simulink model "QBot2_SINGLE_ROBOT_FINDFOLLOW_5_clock_working"  (R2014a)
settings: Solver=ode1  StartTime=0.0  StopTime=inf  FixedStep=0.01  RelTol=1e-3
values from neighbouring files (symbols this model uses):
  x = [0 0 0 0 0 0 0 0 0 0 0 0 ... (23417 elements, 23417x1)]    [plot_data.mat]
undefined symbols (not defined in the file or in its folder): HIL, Kinect, qc_get_step_size
libraries: quarc_library x8
settings Model: SimulationMode=external  CovSFcnEnable=on  ExtModeTrigDuration=10000  Creator=drmadill  LastModifiedBy=student
settings SolverCC: PositivePriorityOrder=on
settings DataIOCC: SignalLoggingSaveFormat=ModelDataLogs
settings OptimizationCC: ExpressionDepthLimit=2147483647
settings DebuggingCC: UnderspecifiedInitializationDetection=Classic  FcnCallInpInsideContextMsg=UseLocalSettings  FrameProcessingCompatibilityMsg=error  StateNameClashWarn=warning
settings RTWCC: SystemTargetFile=quarc_linux_duovero.tlc  TemplateMakefile=quarc_linux_duovero_tmf  Description=QUARC Linux DuoVero Target  ProcessScript=quarc_linux_duovero_make_rtw_hook
settings STFCustomTargetCC: TargetLibSuffix=.a  TargetPreCompLibLocation=C:\PROGRA~3\QUARC\lib\2014a\LINUX_~3\release  CPPClassGenCompliant=on  SystemTargetFile=quarc_linux_duovero.tlc
settings GRTTargetCC: TargetLibSuffix=.a  TargetPreCompLibLocation=C:\PROGRA~3\QUARC\lib\2014a\LINUX_~3\release  ParMdlRefBuildCompliant=off  CompOptLevelCompliant=off  CombineOutputUpdateFcns=off  MatFileLogging=off  GRTInterface=on  ExtMode=on  ExtModeMexFile=quarc_comm  ExtModeMexArgs='-w -d /tmp -uri %u', 'tcpip://192.168.2.49:17001'

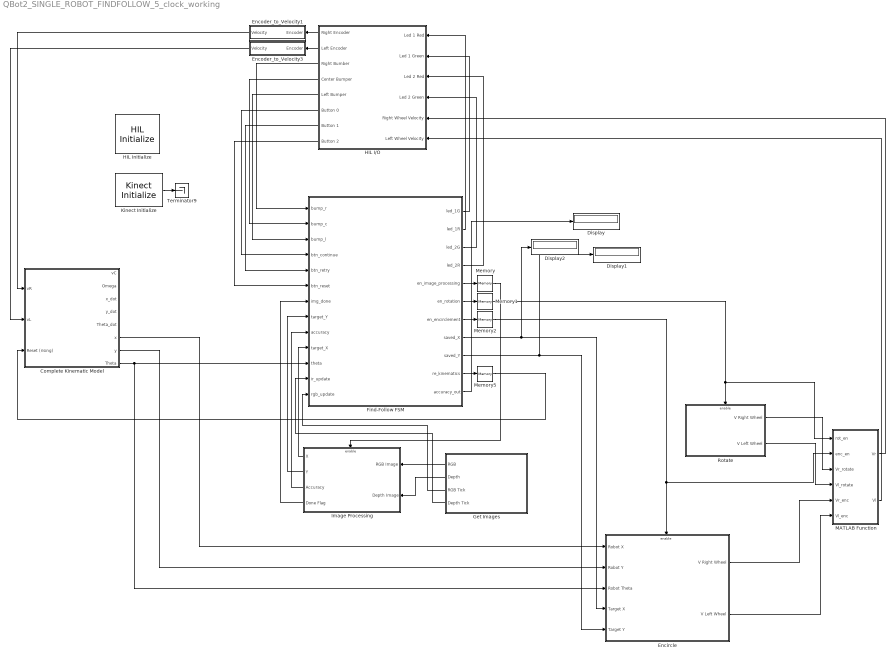
== system QBot2_SINGLE_ROBOT_FINDFOLLOW_5_clock_working ==
  Complete Kinematic Model : Subsystem
  Display : Display
  Display1 : Display
  Display2 : Display
  Encircle : Subsystem  TreatAsAtomicUnit=on
  Encoder_to_Velocity1 : Subsystem
  Encoder_to_Velocity3 : Subsystem
  Find-Follow FSM : Stateflow chart  TreatAsAtomicUnit=on
  Get Images : Subsystem
  HIL I/O : Subsystem
  HIL Initialize : quarc_library/Data Acquisition/Generic/Configuration/HIL Initialize  Priority=-99  object_name=HIL-1  board_type=qbot2  board_number=0  board_options=enc0_dir=0;enc0_filter=1;enc0_a=0;enc0_b=0;enc0_z=1;enc0_reload=0;enc1_dir=0;enc1_filter=1;enc1_a=0;enc1_b=0;enc1_z=1;enc1_reload=0;pwm0_immediate=0;pwm1_immediate=0;pwm2_immediate=0;pwm3_immediate=0;  exclusive=off  active=off  hardware_clocks=[]  clock_modes=[]  initial_clock_frequencies=[]  set_clock_params_at_start=off  set_clock_params_at_switch_in=off  set_clock_frequencies_at_start=off  set_clock_frequencies_at_switch_in=off  analog_input_channels=[0:9]  analog_input_maximums=[5 5 5 5 16.5 3.3 3.3 3.3 3.3]  analog_input_minimums=[0 0 0 0 0 0 0 0 0]  set_analog_input_params_at_start=off  set_analog_input_params_at_switch_in=off  analog_output_channels=[]  analog_output_maximums=[]  analog_output_minimums=[]  initial_analog_outputs=[]  final_analog_outputs=[]  watchdog_analog_outputs=[]  set_analog_output_params_at_start=off  set_analog_output_params_at_switch_in=off  set_analog_outputs_at_start=off  set_analog_outputs_at_switch_in=off  set_analog_outputs_at_terminate=off  set_analog_outputs_at_switch_out=off  set_analog_outputs_on_watchdog=off  digital_input_channels=[8:10 16:18]  digital_output_channels=[11:12 9:10]  digital_output_configuration=[]  initial_digital_outputs=[0]  final_digital_outputs=[0]  watchdog_digital_outputs=[0]  set_digital_output_params_at_start=off  set_digital_output_params_at_switch_in=off  set_digital_outputs_at_start=on  set_digital_outputs_at_switch_in=off  set_digital_outputs_at_terminate=on  set_digital_outputs_at_switch_out=off  set_digital_outputs_on_watchdog=on  encoder_channels=[0:3]  quadrature=[4]  encoder_filter_frequency=[]  initial_encoder_counts=[0]  set_encoder_params_at_start=on  set_encoder_params_at_switch_in=off  set_encoder_counts_at_start=on  set_encoder_counts_at_switch_in=off  pwm_channels=[0:3]  pwm_modes=[0]  pwm_frequency=[20e6/1024]  pwm_configuration=[0]  pwm_alignment=[0]  pwm_polarity=[1]  pwm_leading_deadband=[0]  pwm_trailing_deadband=[0]  initial_pwm_outputs=[0]  final_pwm_outputs=[0]  watchdog_pwm_outputs=[0]  set_pwm_params_at_start=on  set_pwm_params_at_switch_in=off  set_pwm_outputs_at_start=on  set_pwm_outputs_at_switch_in=off  set_pwm_outputs_at_terminate=on  set_pwm_outputs_at_switch_out=off  set_pwm_outputs_on_watchdog=on  other_output_channels=[2000:2001 14000 16000]  initial_other_outputs=[0 0 0 7]  final_other_outputs=[0 0 0 7]  watchdog_other_outputs=[]  set_other_outputs_at_start=on  set_other_outputs_at_switch_in=off  set_other_outputs_at_terminate=on  set_other_outputs_at_switch_out=off  set_other_outputs_on_watchdog=off
  Image Processing : Subsystem
  Kinect Initialize : quarc_library/Multimedia/Kinect Initialize  object_name=Kinect-1  kinect_type=Kinect for XBox 360  identifier=0  sample_time=qc_get_step_size * ceil(0.033 / qc_get_step_size)  active=on
  MATLAB Function : MATLAB Function  TreatAsAtomicUnit=on
  Memory{,1..2,5} (4 alike) : Memory
  Rotate : Subsystem  TreatAsAtomicUnit=on
  Terminator9 : Terminator
  wires:
  Find-Follow FSM/5(en_image_processing) -> Memory/1
  Find-Follow FSM/6(en_rotation) -> Memory1/1
  Find-Follow FSM/7(en_encirclement) -> Memory2/1
  Encoder_to_Velocity3/1(Velocity) -> Complete Kinematic Model/2(vL)
  Encoder_to_Velocity1/1(Velocity) -> Complete Kinematic Model/1(vR)
  Complete Kinematic Model/8(Theta) -> Encircle/3(Robot Theta), Find-Follow FSM/11(theta)
  HIL I/O/1(Right Encoder) -> Encoder_to_Velocity1/1(Encoder)
  HIL I/O/2(Left Encoder) -> Encoder_to_Velocity3/1(Encoder)
  HIL I/O/3(Right Bumber) -> Find-Follow FSM/1(bump_r)
  HIL I/O/4(Center Bumper) -> Find-Follow FSM/2(bump_c)
  HIL I/O/5(Left Bumper) -> Find-Follow FSM/3(bump_l)
  HIL I/O/6(Button 0) -> Find-Follow FSM/4(btn_continue)
  HIL I/O/7(Button 1) -> Find-Follow FSM/5(btn_retry)
  HIL I/O/8(Button 2) -> Find-Follow FSM/6(btn_reset)
  Find-Follow FSM/1(led_1G) -> HIL I/O/2(Led 1 Green)
  Find-Follow FSM/2(led_1R) -> HIL I/O/1(Led 1 Red)
  Find-Follow FSM/3(led_2G) -> HIL I/O/4(Led 2 Green)
  Find-Follow FSM/4(led_2R) -> HIL I/O/3(Led 2 Red)
  MATLAB Function/1(Vr) -> HIL I/O/5(Right Wheel Velocity)
  MATLAB Function/2(Vl) -> HIL I/O/6(Left Wheel Velocity)
  Get Images/1(RGB) -> Image Processing/1(RGB Image)
  Get Images/2(Depth) -> Image Processing/2(Depth Image)
  Get Images/3(RGB Tick) -> Find-Follow FSM/13(rgb_update)
  Get Images/4(Depth Tick) -> Find-Follow FSM/12(ir_update)
  Memory/1 -> Image Processing/Enable
  Image Processing/1(X) -> Find-Follow FSM/10(target_X)
  Image Processing/2(Y) -> Find-Follow FSM/8(target_Y)
  Image Processing/3(Accuracy) -> Find-Follow FSM/9(accuracy)
  Image Processing/4(Done Flag) -> Find-Follow FSM/7(img_done)
  Find-Follow FSM/10(re_kinematics) -> Memory5/1
  Memory1/1 -> MATLAB Function/1(rot_en), Rotate/Enable
  Memory2/1 -> Encircle/Enable, MATLAB Function/2(enc_en)
  Encircle/1(V Right Wheel) -> MATLAB Function/5(Vr_enc)
  Rotate/1(V Right Wheel) -> MATLAB Function/3(Vr_rotate)
  Rotate/2(V Left Wheel) -> MATLAB Function/4(Vl_rotate)
  Encircle/2(V Left Wheel) -> MATLAB Function/6(Vl_enc)
  Find-Follow FSM/8(saved_X) -> Display2/1, Encircle/4(Target X)
  Find-Follow FSM/9(saved_Y) -> Display1/1, Encircle/5(Target Y)
  Complete Kinematic Model/6(x) -> Encircle/1(Robot X)
  Complete Kinematic Model/7(y) -> Encircle/2(Robot Y)
  Memory5/1 -> Complete Kinematic Model/3(Reset (rising))
  Kinect Initialize/1 -> Terminator9/1
  Find-Follow FSM/11(accuracy_out) -> Display/1

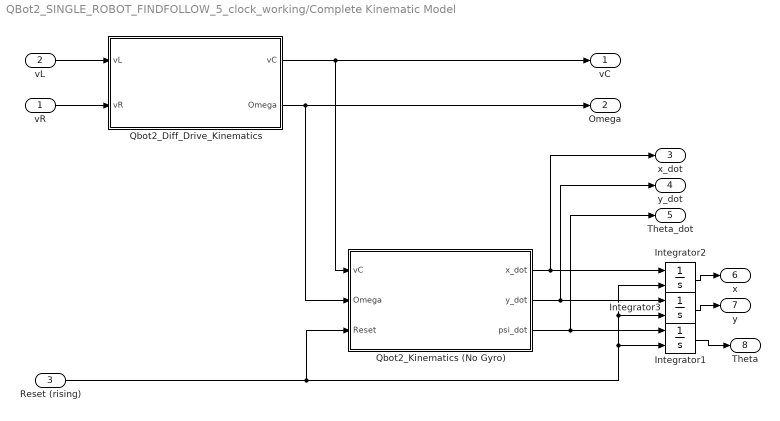
== system QBot2_SINGLE_ROBOT_FINDFOLLOW_5_clock_working/Complete Kinematic Model ==
  vR : Inport
  vL : Inport  Port=2
  Reset (rising) : Inport  Port=3
  Integrator1 : Integrator  ExternalReset=rising
  Integrator2 : Integrator  ExternalReset=rising
  Integrator3 : Integrator  ExternalReset=rising
  Qbot2_Diff_Drive_Kinematics : Subsystem
  Qbot2_Kinematics (No Gyro) : Subsystem
  vC : Outport
  Omega : Outport  Port=2
  x_dot : Outport  Port=3
  y_dot : Outport  Port=4
  Theta_dot : Outport  Port=5
  x : Outport  Port=6
  y : Outport  Port=7
  Theta : Outport  Port=8
  wires:
  Qbot2_Diff_Drive_Kinematics/2(Omega) -> Omega/1, Qbot2_Kinematics (No Gyro)/2(Omega)
  Integrator3/1 -> y/1
  Integrator2/1 -> x/1
  vR/1 -> Qbot2_Diff_Drive_Kinematics/2(vR)
  vL/1 -> Qbot2_Diff_Drive_Kinematics/1(vL)
  Qbot2_Diff_Drive_Kinematics/1(vC) -> vC/1, Qbot2_Kinematics (No Gyro)/1(vC)
  Qbot2_Kinematics (No Gyro)/2(y_dot) -> Integrator3/1, y_dot/1
  Qbot2_Kinematics (No Gyro)/1(x_dot) -> Integrator2/1, x_dot/1
  Qbot2_Kinematics (No Gyro)/3(psi_dot) -> Integrator1/1, Theta_dot/1
  Integrator1/1 -> Theta/1
  Reset (rising)/1 -> Qbot2_Kinematics (No Gyro)/3(Reset), Integrator1/2, Integrator3/2, Integrator2/2

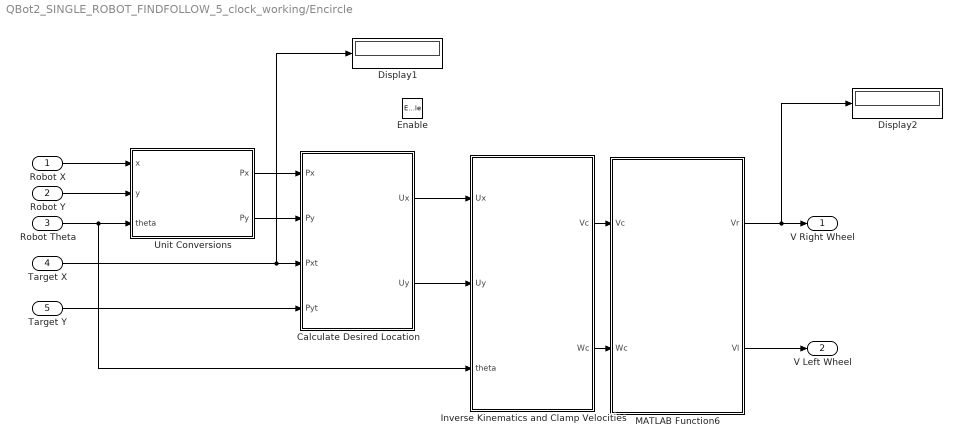
== system QBot2_SINGLE_ROBOT_FINDFOLLOW_5_clock_working/Encircle ==
  Robot X : Inport
  Robot Y : Inport  Port=2
  Robot Theta : Inport  Port=3
  Target X : Inport  Port=4
  Target Y : Inport  Port=5
  Enable : EnablePort
  Calculate Desired Location : MATLAB Function  TreatAsAtomicUnit=on
  Display1 : Display
  Display2 : Display
  Inverse Kinematics and Clamp Velocities : MATLAB Function  TreatAsAtomicUnit=on
  MATLAB Function6 : MATLAB Function  TreatAsAtomicUnit=on
  Unit Conversions : MATLAB Function  TreatAsAtomicUnit=on
  V Right Wheel : Outport  OutputWhenDisabled=reset  InitialOutput=0
  V Left Wheel : Outport  Port=2  OutputWhenDisabled=reset  InitialOutput=0
  wires:
  Calculate Desired Location/2(Uy) -> Inverse Kinematics and Clamp Velocities/2(Uy)
  Calculate Desired Location/1(Ux) -> Inverse Kinematics and Clamp Velocities/1(Ux)
  Target Y/1 -> Calculate Desired Location/4(Pyt)
  Robot X/1 -> Unit Conversions/1(x)
  Unit Conversions/2(Py) -> Calculate Desired Location/2(Py)
  Target X/1 -> Display1/1, Calculate Desired Location/3(Pxt)
  Unit Conversions/1(Px) -> Calculate Desired Location/1(Px)
  Robot Y/1 -> Unit Conversions/2(y)
  Robot Theta/1 -> Inverse Kinematics and Clamp Velocities/3(theta), Unit Conversions/3(theta)
  Inverse Kinematics and Clamp Velocities/1(Vc) -> MATLAB Function6/1(Vc)
  Inverse Kinematics and Clamp Velocities/2(Wc) -> MATLAB Function6/2(Wc)
  MATLAB Function6/1(Vr) -> Display2/1, V Right Wheel/1
  MATLAB Function6/2(Vl) -> V Left Wheel/1

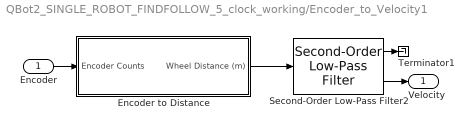
== system QBot2_SINGLE_ROBOT_FINDFOLLOW_5_clock_working/Encoder_to_Velocity1 ==
  Encoder : Inport
  Encoder to Distance : Subsystem
  Second-Order Low-Pass Filter2 : quarc_library/Continuous/Second-Order Low-Pass Filter  params_source=Internal (dialog parameters)  input_width=10  input_zeta=1  input_init=0
  Terminator1 : Terminator
  Velocity : Outport
  wires:
  Second-Order Low-Pass Filter2/2 -> Velocity/1
  Encoder/1 -> Encoder to Distance/1(Encoder Counts)
  Encoder to Distance/1(Wheel Distance (m)) -> Second-Order Low-Pass Filter2/1
  Second-Order Low-Pass Filter2/1 -> Terminator1/1

== system QBot2_SINGLE_ROBOT_FINDFOLLOW_5_clock_working/Encoder_to_Velocity3 ==
  Encoder : Inport
  Encoder to Distance : Subsystem
  Second-Order Low-Pass Filter2 : quarc_library/Continuous/Second-Order Low-Pass Filter  params_source=Internal (dialog parameters)  input_width=10  input_zeta=1  input_init=0
  Terminator1 : Terminator
  Velocity : Outport
  wires:
  Second-Order Low-Pass Filter2/2 -> Velocity/1
  Encoder/1 -> Encoder to Distance/1(Encoder Counts)
  Encoder to Distance/1(Wheel Distance (m)) -> Second-Order Low-Pass Filter2/1
  Second-Order Low-Pass Filter2/1 -> Terminator1/1

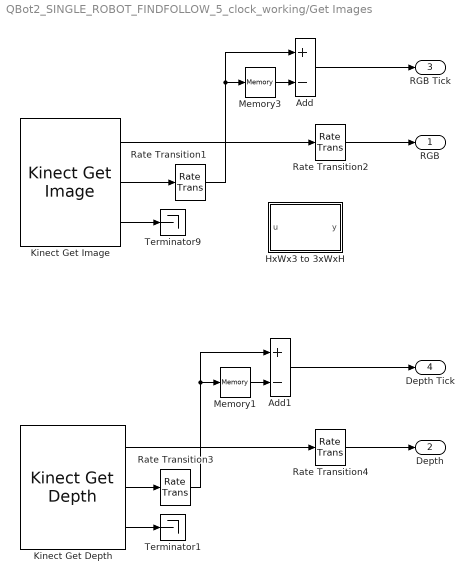
== system QBot2_SINGLE_ROBOT_FINDFOLLOW_5_clock_working/Get Images ==
  Add : Sum  Inputs=+-  OutDataTypeStr=double
  Add1 : Sum  Inputs=+-  OutDataTypeStr=double
  HxWx3 to 3xWxH : MATLAB Function  TreatAsAtomicUnit=on
  Kinect Get Depth : quarc_library/Multimedia/Kinect Get Depth  object_name=Kinect-1  resolution=640 x 480  sample_time=qc_get_step_size * ceil(0.03 / qc_get_step_size)  show_player=off
  Kinect Get Image : quarc_library/Multimedia/Kinect Get Image  object_name=Kinect-1  sensor_type=color  resolution=640 x 480  output_format=MATLAB RGB (HxWx3)  data_type=uint8  backlight=average brightness  flicker=none  brightness=0.2156  gain=1.0  gamma=2.2  autoexposure=on  exposure=0  contrast=1.0  sharpness=0.5  hue=0.0  saturation=1.0  autobalance=on  balance=2700  frame_interval=0  sample_time=qc_get_step_size * ceil(0.03/ qc_get_step_size)
  Memory1 : Memory  InheritSampleTime=on
  Memory3 : Memory  InheritSampleTime=on
  Rate Transition{1..4} (4 alike) : RateTransition
  Terminator1 : Terminator
  Terminator9 : Terminator
  RGB : Outport
  Depth : Outport  Port=2
  RGB Tick : Outport  Port=3
  Depth Tick : Outport  Port=4
  wires:
  Kinect Get Image/1 -> Rate Transition2/1
  Kinect Get Image/3 -> Terminator9/1
  Rate Transition2/1 -> RGB/1
  Kinect Get Image/2 -> Rate Transition1/1
  Add/1 -> RGB Tick/1
  Memory3/1 -> Add/2
  Kinect Get Depth/1 -> Rate Transition4/1
  Kinect Get Depth/3 -> Terminator1/1
  Rate Transition4/1 -> Depth/1
  Kinect Get Depth/2 -> Rate Transition3/1
  Add1/1 -> Depth Tick/1
  Memory1/1 -> Add1/2
  Rate Transition1/1 -> Add/1, Memory3/1
  Rate Transition3/1 -> Add1/1, Memory1/1

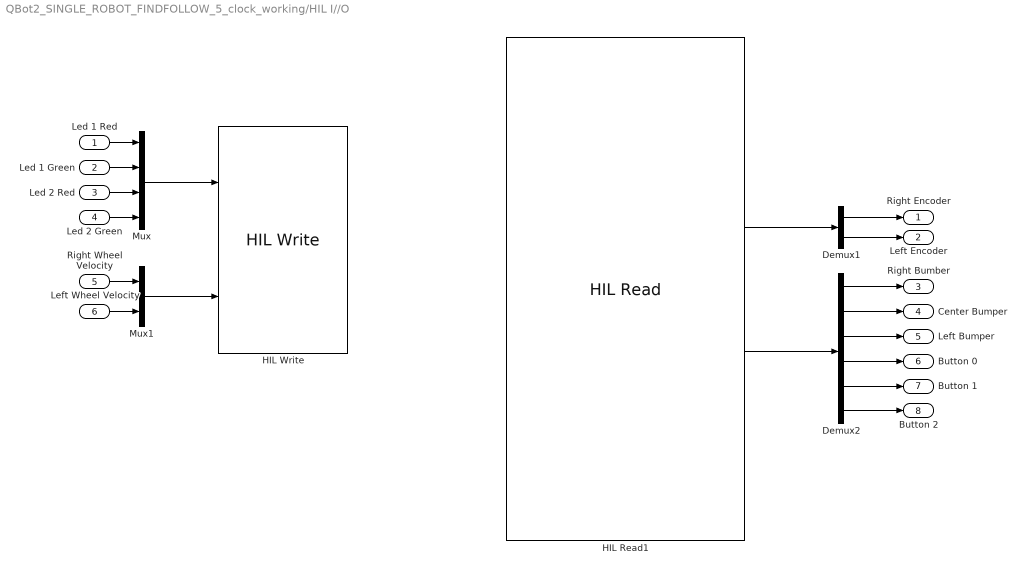
== system QBot2_SINGLE_ROBOT_FINDFOLLOW_5_clock_working/HIL I//O ==
  Led 1 Red : Inport
  Led 1 Green : Inport  Port=2
  Led 2 Red : Inport  Port=3
  Led 2 Green : Inport  Port=4
  Right Wheel Velocity : Inport  Port=5
  Left Wheel Velocity : Inport  Port=6
  Demux1 : Demux  Outputs=2
  Demux2 : Demux  Outputs=6
  HIL Read1 : quarc_library/Data Acquisition/Generic/Immediate I//O/HIL Read  object_name=HIL-1  analog_channels=[4]  encoder_channels=[2 3]  digital_channels=[8:10 16:18]  other_channels=[1002]  sample_time=qc_get_step_size  active=on  vector_output=on  data_type_mode=Inherit via back propagation  encoder_data_type=double  digital_data_type=boolean
  HIL Write : quarc_library/Data Acquisition/Generic/Immediate I//O/HIL Write  object_name=HIL-1  analog_channels=[]  pwm_channels=[]  digital_channels=[9:12]  other_channels=[2000:2001]  sample_time=-1  active=on  vector_input=on
  Mux : Mux
  Mux1 : Mux  Inputs=2
  Right Encoder : Outport
  Left Encoder : Outport  Port=2
  Right Bumber : Outport  Port=3
  Center Bumper : Outport  Port=4
  Left Bumper : Outport  Port=5
  Button 0 : Outport  Port=6
  Button 1 : Outport  Port=7
  Button 2 : Outport  Port=8
  wires:
  HIL Read1/3 -> Demux2/1
  HIL Read1/2 -> Demux1/1
  Demux2/1 -> Right Bumber/1
  Demux2/2 -> Center Bumper/1
  Demux2/3 -> Left Bumper/1
  Demux2/4 -> Button 0/1
  Demux2/5 -> Button 1/1
  Demux2/6 -> Button 2/1
  Mux1/1 -> HIL Write/2
  Mux/1 -> HIL Write/1
  Led 1 Red/1 -> Mux/1
  Led 1 Green/1 -> Mux/2
  Led 2 Red/1 -> Mux/3
  Led 2 Green/1 -> Mux/4
  Right Wheel Velocity/1 -> Mux1/1
  Left Wheel Velocity/1 -> Mux1/2
  Demux1/1 -> Right Encoder/1
  Demux1/2 -> Left Encoder/1

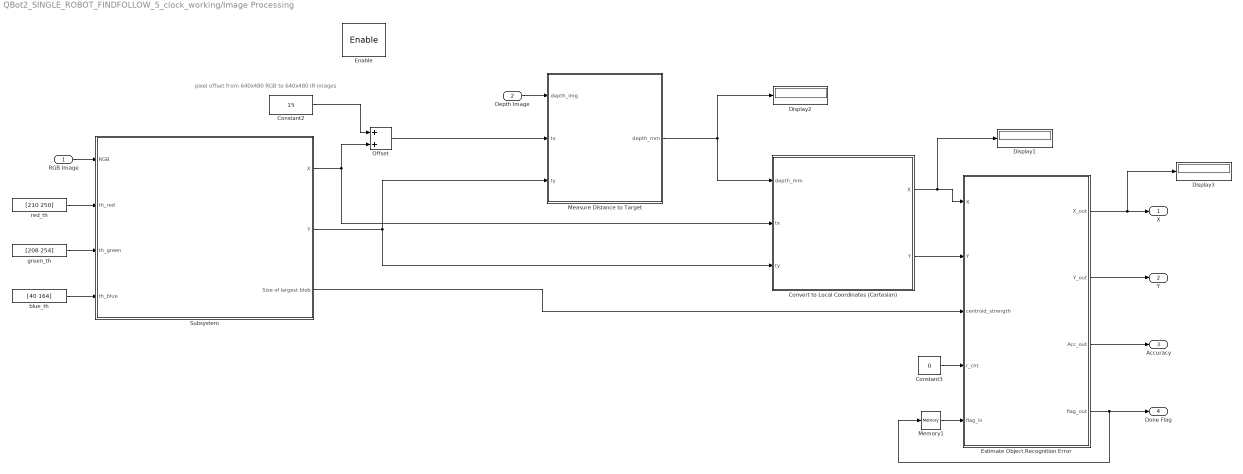
== system QBot2_SINGLE_ROBOT_FINDFOLLOW_5_clock_working/Image Processing ==
  note: pixel offset from 640x480 RGB to 640x480 IR images
  RGB Image : Inport
  Depth Image : Inport  Port=2
  Enable : EnablePort
  Constant2 : Constant  Value=15
  Constant3 : Constant  Value=0
  Convert to Local Coordinates (Cartesian) : MATLAB Function  TreatAsAtomicUnit=on
  Display1 : Display
  Display2 : Display
  Display3 : Display
  Estimate Object Recognition Error : MATLAB Function  TreatAsAtomicUnit=on
  Measure Distance to Target : MATLAB Function  TreatAsAtomicUnit=on
  Memory1 : Memory  X0=1
  Offset : Sum
  Subsystem : Subsystem
  blue_th : Constant  Value=[40 164]
  green_th : Constant  Value=[208 254]
  red_th : Constant  Value=[210 250]
  X : Outport
  Y : Outport  Port=2
  Accuracy : Outport  Port=3
  Done Flag : Outport  Port=4  OutDataTypeStr=boolean
  wires:
  red_th/1 -> Subsystem/2(th_red)
  Measure Distance to Target/1(depth_mm) -> Convert to Local Coordinates (Cartesian)/1(depth_mm), Display2/1
  green_th/1 -> Subsystem/3(th_green)
  blue_th/1 -> Subsystem/4(th_blue)
  Depth Image/1 -> Measure Distance to Target/1(depth_img)
  Subsystem/1(X) -> Offset/2, Convert to Local Coordinates (Cartesian)/2(tx)
  Subsystem/3(Size of largest blob) -> Estimate Object Recognition Error/3(centroid_strength)
  RGB Image/1 -> Subsystem/1(RGB)
  Subsystem/2(Y) -> Measure Distance to Target/3(ty), Convert to Local Coordinates (Cartesian)/3(ty)
  Convert to Local Coordinates (Cartesian)/2(Y) -> Estimate Object Recognition Error/2(Y)
  Memory1/1 -> Estimate Object Recognition Error/5(flag_in)
  Estimate Object Recognition Error/1(X_out) -> Display3/1, X/1
  Estimate Object Recognition Error/3(Acc_out) -> Accuracy/1
  Estimate Object Recognition Error/4(flag_out) -> Done Flag/1, Memory1/1
  Convert to Local Coordinates (Cartesian)/1(X) -> Display1/1, Estimate Object Recognition Error/1(X)
  Constant2/1 -> Offset/1
  Offset/1 -> Measure Distance to Target/2(tx)
  Estimate Object Recognition Error/2(Y_out) -> Y/1
  Constant3/1 -> Estimate Object Recognition Error/4(r_cht)

== system QBot2_SINGLE_ROBOT_FINDFOLLOW_5_clock_working/Rotate ==
  Enable : EnablePort
  Turn by constant velocity : MATLAB Function  TreatAsAtomicUnit=on
  V Right Wheel : Outport  OutputWhenDisabled=reset  InitialOutput=0
  V Left Wheel : Outport  Port=2  OutputWhenDisabled=reset  InitialOutput=0
  wires:
  Turn by constant velocity/1(Vr) -> V Right Wheel/1
  Turn by constant velocity/2(Vl) -> V Left Wheel/1

== system QBot2_SINGLE_ROBOT_FINDFOLLOW_5_clock_working/Complete Kinematic Model/Qbot2_Diff_Drive_Kinematics ==
  vL : Inport
  vR : Inport  Port=2
  Qbot2_Diff_Drive_Kinematics : MATLAB Function  TreatAsAtomicUnit=on
  vC : Outport
  Omega : Outport  Port=2
  wires:
  Qbot2_Diff_Drive_Kinematics/2(Omega) -> Omega/1
  vR/1 -> Qbot2_Diff_Drive_Kinematics/2(vR)
  Qbot2_Diff_Drive_Kinematics/1(vC) -> vC/1
  vL/1 -> Qbot2_Diff_Drive_Kinematics/1(vL)

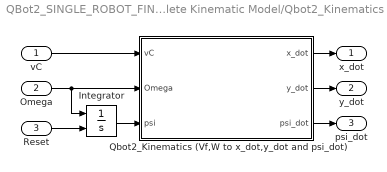
== system QBot2_SINGLE_ROBOT_FINDFOLLOW_5_clock_working/Complete Kinematic Model/Qbot2_Kinematics (No Gyro) ==
  vC : Inport
  Omega : Inport  Port=2
  Reset : Inport  Port=3
  Integrator : Integrator  ExternalReset=rising
  Qbot2_Kinematics (Vf,W to x_dot,y_dot and psi_dot) : MATLAB Function  TreatAsAtomicUnit=on
  x_dot : Outport
  y_dot : Outport  Port=2
  psi_dot : Outport  Port=3
  wires:
  Qbot2_Kinematics (Vf,W to x_dot,y_dot and psi_dot)/2(y_dot) -> y_dot/1
  Omega/1 -> Qbot2_Kinematics (Vf,W to x_dot,y_dot and psi_dot)/2(Omega), Integrator/1
  Qbot2_Kinematics (Vf,W to x_dot,y_dot and psi_dot)/1(x_dot) -> x_dot/1
  vC/1 -> Qbot2_Kinematics (Vf,W to x_dot,y_dot and psi_dot)/1(vC)
  Integrator/1 -> Qbot2_Kinematics (Vf,W to x_dot,y_dot and psi_dot)/3(psi)
  Qbot2_Kinematics (Vf,W to x_dot,y_dot and psi_dot)/3(psi_dot) -> psi_dot/1
  Reset/1 -> Integrator/2

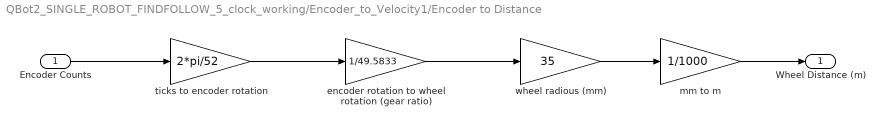
== system QBot2_SINGLE_ROBOT_FINDFOLLOW_5_clock_working/Encoder_to_Velocity1/Encoder to Distance ==
  Encoder Counts : Inport
  " encoder rotation to wheel rotation (gear ratio)" : Gain  Gain=1/49.5833
  mm to m : Gain  Gain=1/1000
  ticks to encoder rotation : Gain  Gain=2*pi/52
  wheel radious (mm) : Gain  Gain=35
  Wheel Distance (m) : Outport
  wires:
  mm to m/1 -> Wheel Distance (m)/1
  wheel radious (mm)/1 -> mm to m/1
  " encoder rotation to wheel rotation (gear ratio)"/1 -> wheel radious (mm)/1
  ticks to encoder rotation/1 -> " encoder rotation to wheel rotation (gear ratio)"/1
  Encoder Counts/1 -> ticks to encoder rotation/1

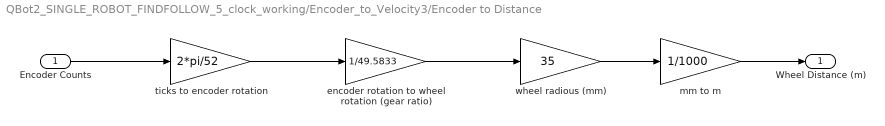
== system QBot2_SINGLE_ROBOT_FINDFOLLOW_5_clock_working/Encoder_to_Velocity3/Encoder to Distance ==
  Encoder Counts : Inport
  " encoder rotation to wheel rotation (gear ratio)" : Gain  Gain=1/49.5833
  mm to m : Gain  Gain=1/1000
  ticks to encoder rotation : Gain  Gain=2*pi/52
  wheel radious (mm) : Gain  Gain=35
  Wheel Distance (m) : Outport
  wires:
  mm to m/1 -> Wheel Distance (m)/1
  wheel radious (mm)/1 -> mm to m/1
  " encoder rotation to wheel rotation (gear ratio)"/1 -> wheel radious (mm)/1
  ticks to encoder rotation/1 -> " encoder rotation to wheel rotation (gear ratio)"/1
  Encoder Counts/1 -> ticks to encoder rotation/1

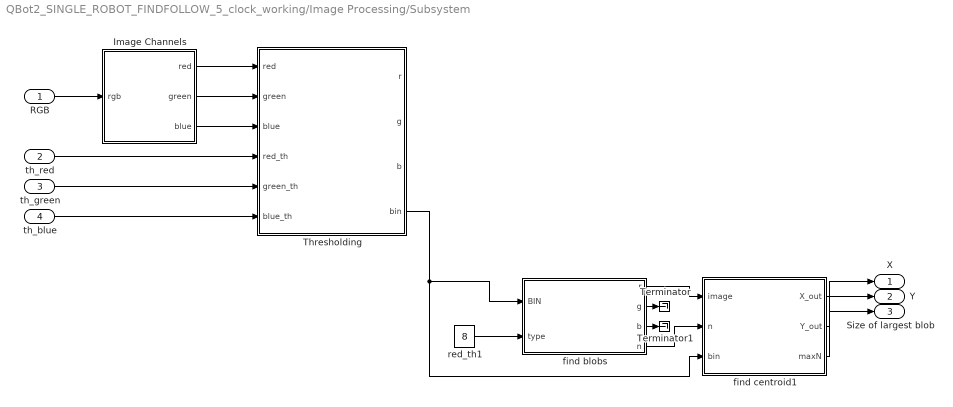
== system QBot2_SINGLE_ROBOT_FINDFOLLOW_5_clock_working/Image Processing/Subsystem ==
  RGB : Inport
  th_red : Inport  Port=2
  th_green : Inport  Port=3
  th_blue : Inport  Port=4
  Image Channels : Subsystem
  Terminator : Terminator
  Terminator1 : Terminator
  Thresholding : MATLAB Function  TreatAsAtomicUnit=on
  find blobs : MATLAB Function  TreatAsAtomicUnit=on
  find centroid1 : MATLAB Function  TreatAsAtomicUnit=on
  red_th1 : Constant  Value=8
  X : Outport
  Y : Outport  Port=2
  Size of largest blob : Outport  Port=3
  wires:
  th_red/1 -> Thresholding/4(red_th)
  th_green/1 -> Thresholding/5(green_th)
  th_blue/1 -> Thresholding/6(blue_th)
  Image Channels/2(green) -> Thresholding/2(green)
  red_th1/1 -> find blobs/2(type)
  Thresholding/4(bin) -> find blobs/1(BIN), find centroid1/3(bin)
  find blobs/3(b) -> Terminator1/1
  Image Channels/1(red) -> Thresholding/1(red)
  find blobs/2(g) -> Terminator/1
  Image Channels/3(blue) -> Thresholding/3(blue)
  find centroid1/3(maxN) -> Size of largest blob/1
  RGB/1 -> Image Channels/1(rgb)
  find blobs/4(n) -> find centroid1/2(n)
  find blobs/1(r) -> find centroid1/1(image)
  find centroid1/1(X_out) -> X/1
  find centroid1/2(Y_out) -> Y/1

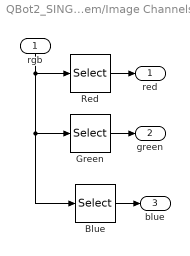
== system QBot2_SINGLE_ROBOT_FINDFOLLOW_5_clock_working/Image Processing/Subsystem/Image Channels ==
  rgb : Inport
  Blue : Selector  NumberOfDimensions=3  InputPortWidth=3  IndexOptions=Select all,Select all,Index vector (dialog)  Indices=1,1,3  OutputSizes=1,1,1
  Green : Selector  NumberOfDimensions=3  InputPortWidth=3  IndexOptions=Select all,Select all,Index vector (dialog)  Indices=1,1,2  OutputSizes=1,1,1
  Red : Selector  NumberOfDimensions=3  InputPortWidth=3  IndexOptions=Select all,Select all,Index vector (dialog)  Indices=[1 3],1,1  OutputSizes=1,1,1
  red : Outport
  green : Outport  Port=2
  blue : Outport  Port=3
  wires:
  rgb/1 -> Red/1, Blue/1, Green/1
  Red/1 -> red/1
  Green/1 -> green/1
  Blue/1 -> blue/1

== matlab function QBot2_SINGLE_ROBOT_FINDFOLLOW_5_clock_working/Image Processing/Convert to Local Coordinates (Cartesian) ==
  data: depth_mm input; tx input; X output; Y output; ty input
% Calculate global coordinates of target object
%
%    ^ +Y
%    |
%    |
%  o  o
% (     ) ------> +X
%  0  0 
%
%
%
% tx,ty : target coordinates on image plane
% depth_mm : distance (not radial distance) to target according to depth image
function [X,Y]  = find_global_coords(depth_mm, tx, ty)
%#codegen
    %RGB_PX_COUNT_HORIZONTAL = 640;
    %RGB_FOV_HORIZONTAL_DEG = 57;
    %RGB_FOV_HORIZONTAL_RAD = 0.99483767363676785884650373803851;
    RGB_DEG_PER_PX_HORIZONTAL = double(0.0015544);
    %X_offset_mm = 14; % distance from RGB camera to center of robot
    %This doesn't work at past 3 Meters cause at 3 meters away the ball is
    %50 pixels big, if its it picks up center at 50-14 = 36. Then it sees
    %the floor
    X_offset_mm = 0;
    HALF_SCREEN_WIDTH_PX = 320;
    
    X = double(depth_mm(:) + X_offset_mm) ./ 1000; % convert to meters
    Y = X .* tan((tx(:) - HALF_SCREEN_WIDTH_PX) .* RGB_DEG_PER_PX_HORIZONTAL);
    
end

== matlab function QBot2_SINGLE_ROBOT_FINDFOLLOW_5_clock_working/Image Processing/Estimate Object Recognition Error ==
  data: X input; X_out output; Y_out output; Acc_out output; Y input; centroid_strength input; r_cht input; flag_out output; flag_in input
% returns a ratio between object dimensions inferred from information given
% by the RGB and IR images.  ratio is between 0 and 1.0
function [X_out, Y_out, Acc_out, flag_out]  = estimate_accuracy(X,Y,centroid_strength,r_cht, flag_in)
%#codegen

if flag_in == true
    flag_out = false;
    X_out = -1;
    Y_out = -1;
    Acc_out = -1;
else
    
    % Ignoring distortion and simplifying the factors of focal length and 
    % aspect ratio to some constant K that will be determined experimentally...
    %
    % u = Kx*X/Z + Ox             (pinhole camera model eq for column position)
    % r_px = u1 - u2 = Kx*(X1-X2)/Z + Ox - Ox
    % X1-X2 = r_actual
    %
    % r_px = Kx*r_actual/Z




    R_ACTUAL_MM = 63.5;     % website listed diameter as 5 inches
    Kx = 463.582;

    [count, ~] = size(X);
    Accuracy = double(zeros(size(X)));

    for i=1:count
        if (centroid_strength(i) == 0 || X(i) == 0)
            Accuracy(i) = 0.0;
        else

            r_px = round((R_ACTUAL_MM * Kx) / X(i));   % infer approximate radius of projected object (in pixels)

            if r_cht == 0
                % Blob Detection used

                area_px = pi * r_px(i) * r_px(i);  % approximate image projection area

                % 0 <= E <= 1.0
                if (area_px > centroid_strength(i))
                    Accuracy(i) = centroid_strength(i) / area_px;
                else
                    Accuracy(i) = area_px / centroid_strength(i);
                end
            else
                % CHT used

                if (r_px > r_cht)
                    Accuracy(i) = r_cht / r_px;
                else
                    Accuracy(i) = r_px / r_cht;
                end
            end
        end
    end
    
    
    % select by max acc instead...
    X_out = X(1);
    Y_out = Y(1);
    %Acc_out = Accuracy(1);
    Acc_out = centroid_strength;
    flag_out = true;
end
    
    
end %end function

== matlab function QBot2_SINGLE_ROBOT_FINDFOLLOW_5_clock_working/MATLAB Function ==
  data: rot_en input; Vr output; enc_en input; Vr_rotate input; Vl_rotate input; Vr_enc input; Vl_enc input; Vl output
function [Vr,Vl] = fcn(rot_en, enc_en, Vr_rotate,Vl_rotate, Vr_enc, Vl_enc )
%#codegen
if rot_en == 1
    Vr = Vr_rotate;
    Vl = Vl_rotate;
elseif enc_en == 1
    Vr = Vr_enc;
    Vl = Vl_enc;
else
   Vr = 0;
   Vl = 0;
end

== stateflow chart QBot2_SINGLE_ROBOT_FINDFOLLOW_5_clock_working/Find-Follow FSM ==
  settings: executeAtInitialization=1
  state InitializeSystem
    entry:
    led_2G = 0;
    led_2R = 0;
    led_1G = 0;
    led_1R = 0;
    en_image_processing = false;
    en_encirclement = false;
    en_rotation = false;
    re_kinematics = 0;
    % dont reset, so we can see what went wrong
    %saved_X = 0;
    %saved_Y = 0;
    %saved_acc = 0;
  state TargetAcquisition
    entry:
    led_1G = 1;
    led_1R = 0;
    exit:
    en_image_processing = false;
    state CentroidFound
      entry:
      led_2G = 1;
      led_2R = 0;
      saved_X = target_X;
      saved_Y = target_Y;
      saved_acc = accuracy;
      accuracy_out = accuracy;
    state ImageProcessingStart
      entry:
      en_image_processing = true;
    state CentroidNotFound
      entry:
      led_2G = 0;
      led_2R = 1;
    (default) -> ImageProcessingStart
    ImageProcessingStart -> (junction 43) : [img_done == true]
    (junction 43) -> CentroidFound [order 1] : [target_X > 0]
    (junction 43) -> CentroidNotFound [order 2]
  state ResetKinematics
    entry:
    re_kinematics = 1;
  state Encirclement
    entry:
    led_1G = 0;
    led_1R = 1;
    led_2G = 0;
    led_2R = 0;
    en_encirclement = true;
    re_kinematics = 0;
    %
    %exit:
  state MoveBeforeSearch
    entry:
    led_1G = 1;
    led_1R = 1;
    new_rgb = 0;
    new_ir = 0;
    state WaitForCameraUpdate
      entry:
      led_2G = 0;
      led_2R = 1;
      %
      during:
      if (rgb_update ~= 0)
      new_rgb = 1;
      end
      if (ir_update ~= 0)
      new_ir = 1;
      end
    state Rotate
      entry:
      en_rotation = true;
      theta_desired = theta + (pi/12);
      %
      exit:
      en_rotation = false;
    Rotate -> WaitForCameraUpdate : [theta >= theta_desired]
  (default) -> InitializeSystem
  Encirclement -> InitializeSystem [order 1] : [btn_reset ~= 0]
  Encirclement -> InitializeSystem [order 2] : after(120, sec)
  InitializeSystem -> TargetAcquisition
  TargetAcquisition -> InitializeSystem : [btn_reset ~= 0]
  CentroidFound -> ResetKinematics [order 1] : [saved_acc > 30]
  ResetKinematics -> Encirclement
  WaitForCameraUpdate -> ImageProcessingStart : [new_rgb == 1 && ...
      |  new_ir == 1]
  CentroidFound -> Rotate [order 2]
  CentroidNotFound -> Rotate
  data: led_1G output; led_1R output; bump_r input; bump_c input; bump_l input; btn_continue input; led_2G output; led_2R output; en_image_processing output boolean; en_rotation output; en_encirclement output; saved_X output; btn_retry input; btn_reset input; img_done input; target_Y input; accuracy input; target_X input; saved_acc local double; saved_Y output; theta input; theta_desired local; re_kinematics output; ir_update input; rgb_update input; new_rgb local; new_ir local; accuracy_out output

== matlab function QBot2_SINGLE_ROBOT_FINDFOLLOW_5_clock_working/Image Processing/Measure Distance to Target ==
  data: depth_img input; depth_mm output; tx input; ty input
function depth_mm  = measure_pixel(depth_img, tx, ty)
%#codegen

[count, ~] = size(tx);
depth_mm = uint16(zeros(size(tx)));

for i = 1:count
    depth_mm(i) = uint16(depth_img(ty(i),tx(i)));
end
end

== matlab function QBot2_SINGLE_ROBOT_FINDFOLLOW_5_clock_working/Image Processing/Subsystem/Thresholding ==
  data: red input; r output; g output; b output; bin output; green input; blue input; red_th input; green_th input; blue_th input
function [r, g, b, bin]  = clr_thr(red, ...
    green, blue, red_th, green_th, blue_th)
% This block supports the Embedded MATLAB subset.
% See the help menu for details. 

red_vec = thresh(red, red_th, 1);

green_vec = thresh(green, green_th, 1);

blue_vec = thresh(blue, blue_th, 1);

tmp = double(and(red_vec, green_vec));
tmp_blob = uint8(and(tmp, blue_vec));
bin = uint8(255*tmp_blob);

% background = uint8(255*double(not(tmp_blob)));
% r = uint8(red.*tmp_blob + background);
% g = uint8(green.*tmp_blob + background);
% b = uint8(blue.*tmp_blob + background);

r = uint8(red.*tmp_blob);
g = uint8(green.*tmp_blob);
b = uint8(blue.*tmp_blob);


return;

%--------------------------------------------------------------------------

function x = thresh(x, th, val)

[row col] = size(x);
for i=1:row
    for j=1:col
        if x(i,j) >= th(1) && x(i, j) <= th(2)
            x(i, j) = val;
        else
            x(i, j) = 0;
        end
    end
end

return;

%--------------------------------------------------------------------------

== matlab function QBot2_SINGLE_ROBOT_FINDFOLLOW_5_clock_working/Image Processing/Subsystem/find blobs ==
  data: BIN input; r output; g output; b output; n output; type input
function [r, g, b, n]  = find_blobs(BIN, type)
% This block supports the Embedded MATLAB subset.
% See the help menu for details. 

idvec = zeros(1, 50);

[ROW COL] = size(BIN);

%{
if ROW>120 || COL>160
    r = uint8(BIN);
    g = uint8(BIN);
    b = uint8(BIN);
    n = -1;
    return;
end
%}

dwnsmple = 4;
row = round(ROW/dwnsmple);
col = round(COL/dwnsmple);
bin = uint8(zeros(row, col));

rw = 0;
% for i=dwnsmple+1:dwnsmple:ROW
for i=1:dwnsmple:ROW
    rw = rw + 1;
    co = 0;
    for j=1:dwnsmple:COL
        co = co + 1;
        bin(rw, co) = uint8(BIN(i, j));
    end
end

% r = uint8(zeros(row, col));
% g = uint8(zeros(row, col));
% b = uint8(zeros(row, col));
r = uint8(bin);
g = uint8(bin);
b = uint8(bin);
n = -1;%count;

% Bin = double(bin)/255;
% binsum = sum(Bin(:));
% ratio = binsum/(row*col);

% if ratio<=0.1
    % Find the 4 or 8 connected reachability matrix
    [eqtable, limg, maxlabel] = find_reachability_matrix(bin, type);
    if maxlabel>=1
        % Find equivalent labels
        table1 = updatetable(eqtable, maxlabel);
        table2 = updatetable2(table1, maxlabel);
        table3 = double(or(table1, table2));
        [idvec, n] = updatetable3(table3, maxlabel);
%     
%     
%         % Label the final image
        Limg = label_image(limg, n, idvec, maxlabel);
        r = uint8(Limg);
        g = uint8(Limg);
        b = uint8(Limg);
    end
%     r = uint8(limg);
%     g = uint8(limg);
%     b = uint8(limg);
% end



return;
%--------------------------------------------------------------------------
function [eqtable, limg, maxlabel] = find_reachability_matrix(img, Type)

[row col] = size(img);

type = Type;
if Type~=4 && Type~=8
    type = 8;
end

% Step 1: Label 8 or 4 connected components
limg = zeros(row, col);
label = 0;
Maxlabel = 50;
for i=1:row
    for j=1:col
        if img(i, j)>0 && limg(i, j)==0
            if (j-1)>=1 && img(i, j-1)>0
                limg(i, j)= limg(i, j-1);
            else
                if label<=(Maxlabel-1)
                    label = label+1;
                    limg(i, j)= label;
                else
                    limg(i, j)= 0;
                end
            end
        end
    end
end

% Find the reachability matrix
maxlabel = label;
eqtable = eye(Maxlabel, Maxlabel);
if maxlabel<1
    return;
end
% eqtable = eye(maxlabel, maxlabel);
for i=2:row
    for j=1:col
        if type == 4
            if img(i, j)>0
                if img(i-1, j)>0 && limg(i, j)~=0
                    eqtable(limg(i, j), limg(i-1, j)) = 1;
                    eqtable(limg(i-1, j), limg(i, j)) = 1;
                end
            end
        elseif type == 8
            if img(i, j)>0 && limg(i, j)~=0
                if (j-1)>=1 && img(i-1, j-1)>0 
                    eqtable(limg(i, j), limg(i-1, j-1)) = 1;
                    eqtable(limg(i-1, j-1), limg(i, j)) = 1;
                end
                if img(i-1, j)>0
                    eqtable(limg(i, j), limg(i-1, j)) = 1;
                    eqtable(limg(i-1, j), limg(i, j)) = 1;
                end
                if (j+1)<=col && img(i-1, j+1)>0
                    eqtable(limg(i, j), limg(i-1, j+1)) = 1;
                    eqtable(limg(i-1, j+1), limg(i, j)) = 1;
                end
            end
        end
        
    end
end

return;
%--------------------------------------------------------------------------
function [table] = updatetable(eqtable, maxlabel)

[row col] = size(eqtable);
table = zeros(row, col);
% etable = eqtable;
for i=1:maxlabel
    tmp1 = eqtable(i, :);
    for j=i+1:maxlabel
        tmp2 = eqtable(j, :);
        iscommon = sum(double(and(tmp1, tmp2)));
        if iscommon
            tmp1 = double(or(tmp1, tmp2));
        end
    end
        table(i, :) = tmp1;
end

return;
%--------------------------------------------------------------------------
function [table] = updatetable2(eqtable, maxlabel)

[row col] = size(eqtable);
table = zeros(row, col);
% etable = eqtable;
for i=maxlabel:-1:1
    tmp1 = eqtable(i, :);
%         i
%         count = count + 1;
%         idvec(i) = count;
    for j=i-1:-1:1
        tmp2 = eqtable(j, :);
        iscommon = sum(double(and(tmp1, tmp2)));
        if iscommon
            tmp1 = double(or(tmp1, tmp2));
%                 find(tmp1==1)
%                 pause
        end
    end
    table(i, :) = tmp1;
end

return;
%--------------------------------------------------------------------------
function [idvec, count] = updatetable3(eqtable, maxlabel)

[row col] = size(eqtable);
table = zeros(row, col);
count = 0;
idvec = zeros(1, col);
% etable = eqtable;
for i=1:maxlabel
    tmp1 = eqtable(i, :);
    if tmp1(i)~=0
        count = count + 1;
        idvec(i) = count;
        for j=i+1:maxlabel
            tmp2 = eqtable(j, :);
            iscommon = sum(double(and(tmp1, tmp2)));
            if iscommon
                tmp1 = double(or(tmp1, tmp2));
            end
        end
        table(i, :) = tmp1;
        for j=i+1:maxlabel
            if tmp1(j)==1
                idvec(j) = count;
                eqtable(j, :) = table(j, :);
            end
        end
    end
end

return;
%--------------------------------------------------------------------------
function [Limg] = label_image(limg, count, idvec, maxlabel)

[row col] = size(limg);
Limg = limg;
for i=1:row
    for j=1:col
        if Limg(i, j)>0 && Limg(i, j)<=maxlabel
%             if count<=255
%                 Limg(i, j) = uint8(round((255/count)*idvec(Limg(i, j))));
%             else
                Limg(i, j) = uint8(idvec(Limg(i, j)));
%             end
        end
    end
end

return;
%--------------------------------------------------------------------------

== matlab function QBot2_SINGLE_ROBOT_FINDFOLLOW_5_clock_working/Image Processing/Subsystem/find centroid1 ==
  data: X_out output; Y_out output; image input; n input; bin input; maxN output
function [X_out, Y_out, maxN]  = find_centroid(image, n, bin)
% This block supports the Embedded MATLAB subset.
% See the help menu for details. 

[binrow bincol] = size(bin);
cr = bin;
cg = bin;
cb = bin;
[row col] = size(image);
x = -1;
y = -1;
maxN = -1;
if n>50
    X_out = -1;
    Y_out = -1;
    return;
end
X = zeros(1, 50);
Y = zeros(1, 50);
N = zeros(1, 50);
for L=1:n
    for i=1:row
        for j=1:col
            if image(i, j) == L
                X(L) = X(L) + j;
                Y(L) = Y(L) + i;
                N(L) = N(L) + 1;
            end
        end
    end
end

%maxN = -1;
maxNid = -1;
for L=1:n
    val = N(L);
    if val > maxN
        maxN = val;
        maxNid = L;
    end
end

if maxN > 0
    x = 4*(X(maxNid)/N(maxNid));
    y = 4*(Y(maxNid)/N(maxNid));
    
    for i=fix(y-2):fix(y+2)
        if i>=1 && i<=binrow
            for j=fix(x-2):fix(x+2) 
                if j>=1 && j<=bincol
                    cr(i, j) = 255;
                    cg(i, j) = 0;
                    cb(i, j) = 0;
                end
            end
        end
    end
    
end

X_out = x;
Y_out = y;

return;
%--------------------------------------------------------------------------

== matlab function QBot2_SINGLE_ROBOT_FINDFOLLOW_5_clock_working/Complete Kinematic Model/Qbot2_Diff_Drive_Kinematics/Qbot2_Diff_Drive_Kinematics ==
  data: vL input; vC output; vR input; Omega output
function [vC,Omega] = fcn(vL,vR)
%#codegen

d= 0.235;

vC=0.5*(vL+vR);
Omega=(1/d)*(vR-vL);

== matlab function QBot2_SINGLE_ROBOT_FINDFOLLOW_5_clock_working/Complete Kinematic Model/Qbot2_Kinematics (No Gyro)/Qbot2_Kinematics (Vf,W to x_dot,y_dot and psi_dot) ==
  data: vC input; x_dot output; Omega input; y_dot output; psi input; psi_dot output
function [x_dot,y_dot,psi_dot] = fcn(vC,Omega,psi)
%#codegen


x_dot=cos(psi)*vC;
y_dot=sin(psi)*vC;
psi_dot= Omega;

== matlab function QBot2_SINGLE_ROBOT_FINDFOLLOW_5_clock_working/Encircle/Calculate Desired Location ==
  data: Px input; Ux output; Py input; Pxt input; Pyt input; Uy output
function [Ux, Uy] = UxUy(Px,Py,Pxt,Pyt)
% pxt, pyt are the target's x and y


%#codegen
%rho_star=.5;
%omega_star=.5;
 
krho = .25/2; % forward v gain
kphi = .5/2;   % 
w_d= 0.1;
 
U = [0 0];
rho_size = 1;
phi_size = 2;
[phi, rho] = cart2pol(Px,Py);
[phi_d, rho_d] = cart2pol(Pxt,Pyt);
 
[phi_dif, rho_dif] = cart2pol((Px-Pxt),(Py-Pyt));
 
PxD = Px - Pxt;
PyD = Py - Pyt;
 
 
 
J_i=[PxD/(sqrt(PxD^2+PyD^2)) PyD/(sqrt(PxD^2+PyD^2)); -PyD/(PxD^2+PyD^2) PxD/(PxD^2+PyD^2)];
 
 
 
 
%J_i=[(Px-Pxt)/phi_dif (Py-Pyt)/phi_dif;...
%    -(Py-Pyt)/((1+((Py-Pyt)/(PD))^2)*(Px-Pxt)^2)  1/((1+((Py-Pyt)/(PD))^2)*(Px-Pxt))];
 
 
 
%J_i=[ (Px-Pxt)/phi (Py-Pyt)/phi_dif;    -(Py-Pyt)/(phi_dif)^2  (Px-Pxt)/(phi_dif)^2 ];
 
rhoi_dot = krho*(rho_size-rho_dif);
%phii_d= phi/2
%phii_d = phi_d - phii_d
phii_dot = w_d; %+ kphi*((phi_size-phi)/2);
V_i= [rhoi_dot; phii_dot];
Rt = [ 1 0; 0 1];
 
 
%U = Rt*(J_i'*V_i);
U = inv(J_i)*V_i; 
Ux = U(1);
Uy = U(2);

== matlab function QBot2_SINGLE_ROBOT_FINDFOLLOW_5_clock_working/Rotate/Turn by constant velocity ==
  data: Vr output; Vl output
function [Vr,Vl] = rotate()
%#codegen
scale = 0.05;

% can only turn left
Vr = scale;
Vl = -scale;

== matlab function QBot2_SINGLE_ROBOT_FINDFOLLOW_5_clock_working/Encircle/Inverse Kinematics and Clamp Velocities ==
  data: Ux input; Vc output; Uy input; theta input; Wc output
function [Vc,Wc] = UxUy2VcWc(Ux, Uy, theta)
VC_MAX = 0.2;
WC_MAX = 0.1;
l=.0235; %#length between the two wheels in meters

kin_inv = inv([cos(theta) -l*sin(theta) ; sin(theta) l*cos(theta)]);
P =  kin_inv*[Ux;Uy];
Vc = P(1);
Wc = P(2);
% 
% if P(1) > VC_MAX
%     Vc = VC_MAX;
% else
%     Vc=P(1);
% end
% 
% if P(2) > WC_MAX
%     Wc = WC_MAX;
% else
%     Wc = P(2);
% end

== matlab function QBot2_SINGLE_ROBOT_FINDFOLLOW_5_clock_working/Encircle/MATLAB Function6 ==
  data: Vc input; Vr output; Wc input; Vl output
function [Vr,Vl] = VcWc2VrVl(Vc,Wc)
%#codegen

l=.0235;
Vr = Vc+(1/2)*(l*2)*Wc;
Vl = Vc-(1/2)*(l*2)*Wc;

== matlab function QBot2_SINGLE_ROBOT_FINDFOLLOW_5_clock_working/Encircle/Unit Conversions ==
  data: x input; Px output; Py output; y input; theta input
function [Px,Py] = PxPy_convert(x, y, theta)
%#codegen

l=.0235; %#length between the two wheels in meters
%R=.0175; %#R or signed distance from ICC (Instanteous center of curvature) in meters
Px= x+l*cos(theta)
Py = y+l*sin(theta)

== matlab function QBot2_SINGLE_ROBOT_FINDFOLLOW_5_clock_working/Get Images/HxWx3 to 3xWxH ==
  data: u input; y output
function y = fcn(u)
%#codegen

y = permute(u, [3 2 1]);
